simulink model "Calc_SubSystem"  (R2018b)
settings: Solver=FixedStepDiscrete  StartTime=0.0  StopTime=10.0  RelTol=1e-3
settings Model: Creator=karim  LastModifiedBy=karim
settings OptimizationCC: DefaultParameterBehavior=Inlined  EnhancedBackFolding=on  PassReuseOutputArgsAs=Individual arguments  OptimizeBlockOrder=speed  DifferentSizesBufferReuse=on  OptimizationCustomize=off
settings DebuggingCC: UnderspecifiedInitializationDetection=Classic  MergeDetectMultiDrivingBlocksExec=none  ParameterTunabilityLossMsg=error
settings ModelReferenceCC: PropagateSignalLabelsOutOfModel=off
settings SFSimCC: MATLABDynamicMemAlloc=off
settings RTWCC: SystemTargetFile=ert.tlc  GenCodeOnly=on  TemplateMakefile=ert_default_tmf  GenerateReport=on  IncludeHyperlinkInReport=on  LaunchReport=on  GenerateTraceInfo=on  GenerateTraceReport=on  GenerateTraceReportSl=on  GenerateTraceReportSf=on  GenerateTraceReportEml=on
settings CodeAppCC: ForceParamTrailComments=on  IgnoreCustomStorageClasses=off  OperatorAnnotations=on  SimulinkDataObjDesc=on  SFDataObjDesc=on  InsertBlockDesc=on
settings ERTTargetCC: TargetLangStandard=C99 (ISO)  GenerateSampleERTMain=on  InlinedParameterPlacement=NonHierarchical  ERTCustomFileTemplate=example_file_process.tlc

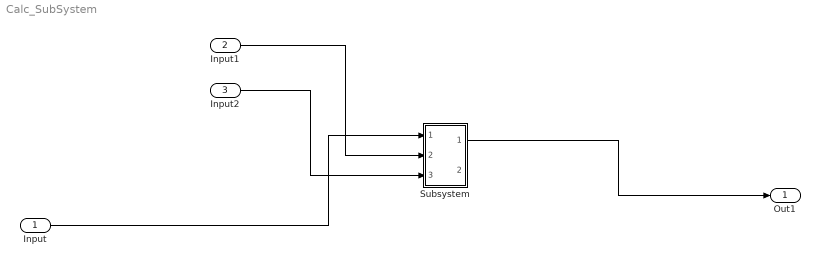
== system Calc_SubSystem ==
  Input : Inport
  Input1 : Inport  Port=2
  Input2 : Inport  Port=3
  Subsystem : Subsystem
  Out1 : Outport
  wires:
  Input/1 -> Subsystem/1(Input)
  Input1/1 -> Subsystem/2(Input1)
  Input2/1 -> Subsystem/3(Input2)
  Subsystem/1(Out1) -> Out1/1

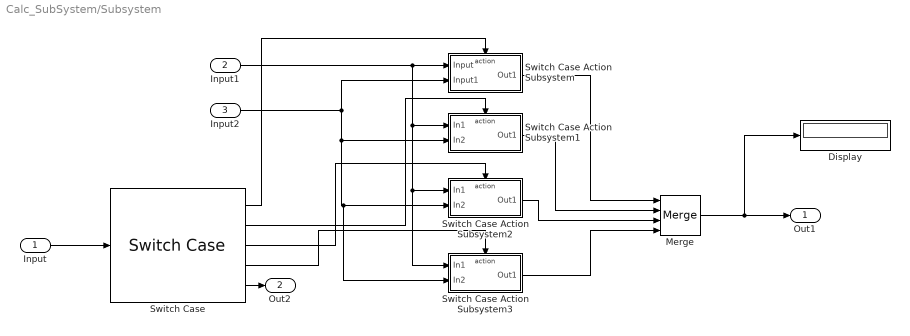
== system Calc_SubSystem/Subsystem ==
  Input : Inport
  Input1 : Inport  Port=2
  Input2 : Inport  Port=3
  Display : Display
  Merge : Merge  Inputs=4
  Switch Case : SwitchCase  CaseConditions={1 , 2 , 3 , 4}
  Switch Case Action Subsystem : Subsystem  TreatAsAtomicUnit=on
  Switch Case Action Subsystem1 : Subsystem  TreatAsAtomicUnit=on
  Switch Case Action Subsystem2 : Subsystem  TreatAsAtomicUnit=on
  Switch Case Action Subsystem3 : Subsystem  TreatAsAtomicUnit=on
  Out1 : Outport
  Out2 : Outport  Port=2
  wires:
  Switch Case/3 -> Switch Case Action Subsystem2/Action
  Switch Case Action Subsystem1/1(Out1) -> Merge/2
  Input2/1 -> Switch Case Action Subsystem/2(Input1), Switch Case Action Subsystem3/2(In2), Switch Case Action Subsystem2/2(In2), Switch Case Action Subsystem1/2(In2)
  Switch Case Action Subsystem3/1(Out1) -> Merge/4
  Merge/1 -> Out1/1, Display/1
  Switch Case/1 -> Switch Case Action Subsystem/Action
  Input1/1 -> Switch Case Action Subsystem3/1(In1), Switch Case Action Subsystem2/1(In1), Switch Case Action Subsystem1/1(In1), Switch Case Action Subsystem/1(Input)
  Switch Case Action Subsystem/1(Out1) -> Merge/1
  Switch Case/2 -> Switch Case Action Subsystem1/Action
  Input/1 -> Switch Case/1
  Switch Case Action Subsystem2/1(Out1) -> Merge/3
  Switch Case/4 -> Switch Case Action Subsystem3/Action
  Switch Case/5 -> Out2/1

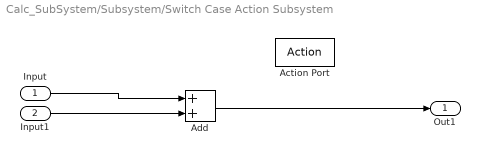
== system Calc_SubSystem/Subsystem/Switch Case Action Subsystem ==
  Input : Inport
  Input1 : Inport  Port=2
  Action Port : ActionPort  ActionType=case
  Add : Sum
  Out1 : Outport
  wires:
  Add/1 -> Out1/1
  Input/1 -> Add/1
  Input1/1 -> Add/2

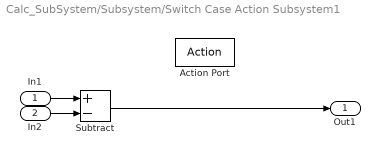
== system Calc_SubSystem/Subsystem/Switch Case Action Subsystem1 ==
  In1 : Inport
  In2 : Inport  Port=2
  Action Port : ActionPort  ActionType=case
  Subtract : Sum  Inputs=+-
  Out1 : Outport
  wires:
  Subtract/1 -> Out1/1
  In1/1 -> Subtract/1
  In2/1 -> Subtract/2

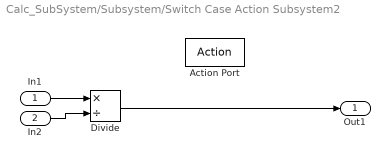
== system Calc_SubSystem/Subsystem/Switch Case Action Subsystem2 ==
  In1 : Inport
  In2 : Inport  Port=2
  Action Port : ActionPort  ActionType=case
  Divide : Product  Inputs=*/
  Out1 : Outport
  wires:
  Divide/1 -> Out1/1
  In1/1 -> Divide/1
  In2/1 -> Divide/2

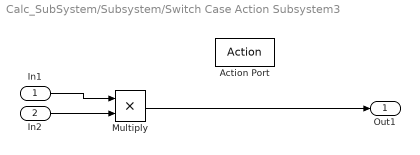
== system Calc_SubSystem/Subsystem/Switch Case Action Subsystem3 ==
  In1 : Inport
  In2 : Inport  Port=2
  Action Port : ActionPort  ActionType=case
  Multiply : Product
  Out1 : Outport
  wires:
  Multiply/1 -> Out1/1
  In2/1 -> Multiply/2
  In1/1 -> Multiply/1
